simulink model "UDPMain_MoveToPoint"  (R2022a)
settings: Solver=FixedStepAuto  StartTime=0.0  StopTime=inf  FixedStep=1/model_frequency  RelTol=1e-3
values from neighbouring files (symbols this model uses):
  markers = [markers;i]    [loadMapData.m]
  send_data_length = num_floats_to_send*4    (= 12)    [initUDP.m]
  steerLim = [-40,40]    [initUDP.m]
  velLim = [-2,5]    [initUDP.m]
libraries: slrealtimeutilitieslib x2, slrealtimeiplib x2, simulink_extras x1
settings Model: Creator=aljaz  LastModifiedBy=aljaz
settings SolverCC: AlgebraicLoopSolver=TrustRegion
settings DebuggingCC: UnconnectedInputMsg=warning  UnconnectedOutputMsg=warning  UnconnectedLineMsg=warning  SFMachineParentedDataDiag=warning
settings RTWCC: DLArmComputeVersion=19.05

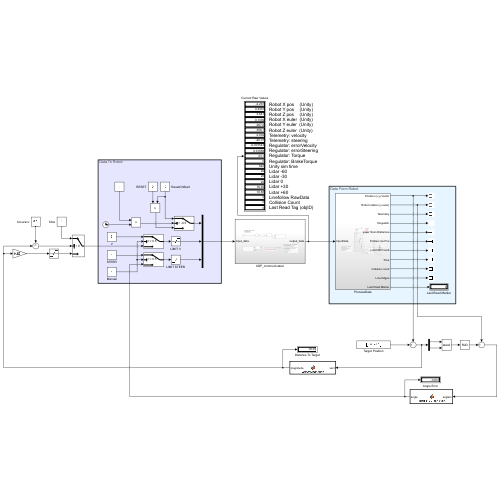
[thumbnail: Simulink's stored preview of the top-level diagram]
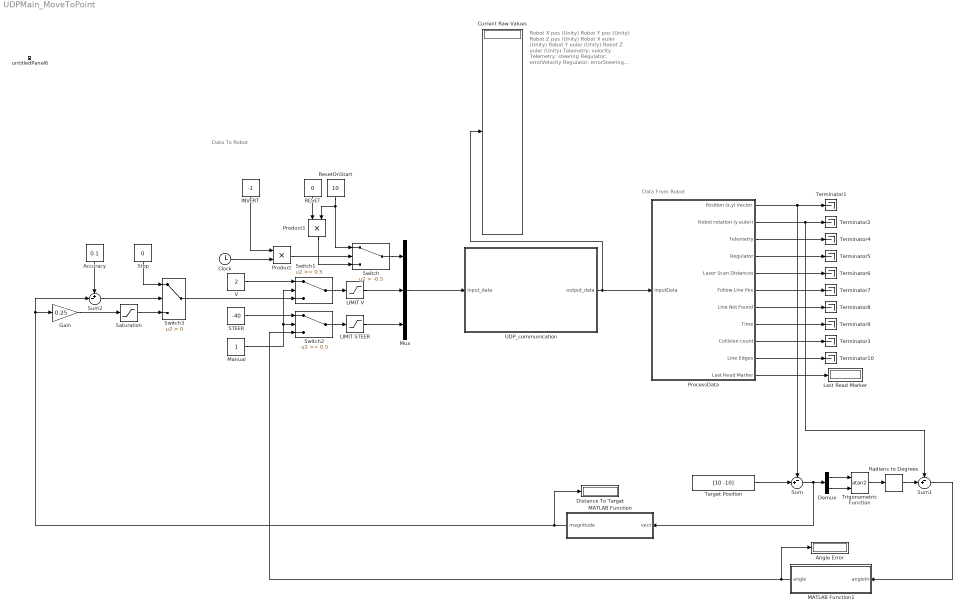
== system UDPMain_MoveToPoint ==
  note: Data From Robot
  note: Data To Robot
  note: Robot X pos (Unity)
      | Robot Y pos (Unity)
      | Robot Z pos (Unity)
      | Robot X euler (Unity)
      | Robot Y euler (Unity)
      | Robot Z euler (Unity)
      | Telemetry: velocity
      | Telemetry: steering
      | Regulator: errorVelocity
      | Regulator: errorSteering
      | Regulator: Torque
      | Regulator: BrakeTorque
      | Unity sim time
      | Lidar -60
      | Lidar -30
      | Lidar 0
      | Lidar +30
      | Lidar +60
      | Linefollow RawData
      | Collision Count
      | Last Read Tag (objID)
  Accuracy : Constant  Value=0.1
  Angle Error : Display
  Clock : Clock
  Current Raw Values : Display
  Demux : Demux  Outputs=2
  Distance To Target : Display
  Gain : Gain  Gain=0.25
  INVERT : Constant  Value=-1
  LIMIT STEER : Saturate  UpperLimit=steerLim(2)  LowerLimit=steerLim(1)
  LIMIT V : Saturate  UpperLimit=velLim(2)  LowerLimit=velLim(1)
  Last Read Marker : Display
  MATLAB Function : MATLAB Function  TreatAsAtomicUnit=on
  MATLAB Function1 : MATLAB Function  TreatAsAtomicUnit=on
  Manual : Constant
  Mux : Mux  Inputs=3
  ProcessData : Subsystem
  Product : Product
  Product1 : Product
  RESET : Constant  Value=0
  Radians to Degrees : simulink_extras/Transformations/Radians to Degrees
  ResetOnStart : Constant  Value=10
  STEER : Constant  Value=-40
  Saturation : Saturate  UpperLimit=1  LowerLimit=-1
  Stop : Constant  Value=0
  Sum : Sum  Inputs=-+|
  Sum1 : Sum  Inputs=-+|
  Sum2 : Sum  Inputs=+-|
  Switch : Switch  Criteria=u2 > Threshold  Threshold=-0.5  SaturateOnIntegerOverflow=off  InputSameDT=off
  Switch1 : Switch  Threshold=0.5  SaturateOnIntegerOverflow=off  InputSameDT=off
  Switch2 : Switch  Threshold=0.5  SaturateOnIntegerOverflow=off  InputSameDT=off
  Switch3 : Switch  Criteria=u2 > Threshold  SaturateOnIntegerOverflow=off  InputSameDT=off
  Target Position : Constant  Value=[10 -10]
  Terminator{1..10} (10 alike) : Terminator
  Trigonometric Function : Trigonometry  Operator=atan2
  UDP_communication : Subsystem
  V : Constant  Value=2
  untitledPanel6 : Subsystem  Tag=HiddenForWebPanel  IsWebBlockPanel=on
  wires:
  UDP_communication/1(output_data) -> Current Raw Values/1, ProcessData/1(InputData)
  ProcessData/9(Collision count) -> Terminator3/1
  ProcessData/2(Robot rotation (y euler)) -> Terminator2/1, Sum1/1
  ProcessData/1(Position (x,y) Vector) -> Sum/1, Terminator1/1
  Mux/1 -> UDP_communication/1(input_data)
  INVERT/1 -> Product/1
  Product/1 -> Switch/2
  Clock/1 -> Product/2
  Switch/1 -> Mux/1
  RESET/1 -> Product1/1
  LIMIT V/1 -> Mux/2
  LIMIT STEER/1 -> Mux/3
  Switch1/1 -> LIMIT V/1
  V/1 -> Switch1/1
  Manual/1 -> Switch2/2, Switch1/2
  Switch2/1 -> LIMIT STEER/1
  STEER/1 -> Switch2/1
  ProcessData/3(Telemetry) -> Terminator4/1
  ProcessData/4(Regulator) -> Terminator5/1
  ProcessData/5(Laser Scan Distances) -> Terminator6/1
  ProcessData/6(Follow Line Pos) -> Terminator7/1
  ProcessData/7(Line Not Found) -> Terminator8/1
  ProcessData/8(Time) -> Terminator9/1
  ResetOnStart/1 -> Switch/1, Product1/2
  Product1/1 -> Switch/3
  ProcessData/11(Last Read Marker) -> Last Read Marker/1
  ProcessData/10(Line Edges) -> Terminator10/1
  Sum1/1 -> MATLAB Function1/1(angleIn)
  Target Position/1 -> Sum/2
  Sum/1 -> MATLAB Function/1(vect), Demux/1
  Demux/1 -> Trigonometric Function/1
  Demux/2 -> Trigonometric Function/2
  Trigonometric Function/1 -> Radians to Degrees/1
  MATLAB Function/1(magnitude) -> Sum2/2, Gain/1, Distance To Target/1
  Gain/1 -> Saturation/1
  Radians to Degrees/1 -> Sum1/2
  Switch3/1 -> Switch1/3
  Sum2/1 -> Switch3/2
  Saturation/1 -> Switch3/3
  Stop/1 -> Switch3/1
  Accuracy/1 -> Sum2/1
  MATLAB Function1/1(angle) -> Switch2/3, Angle Error/1

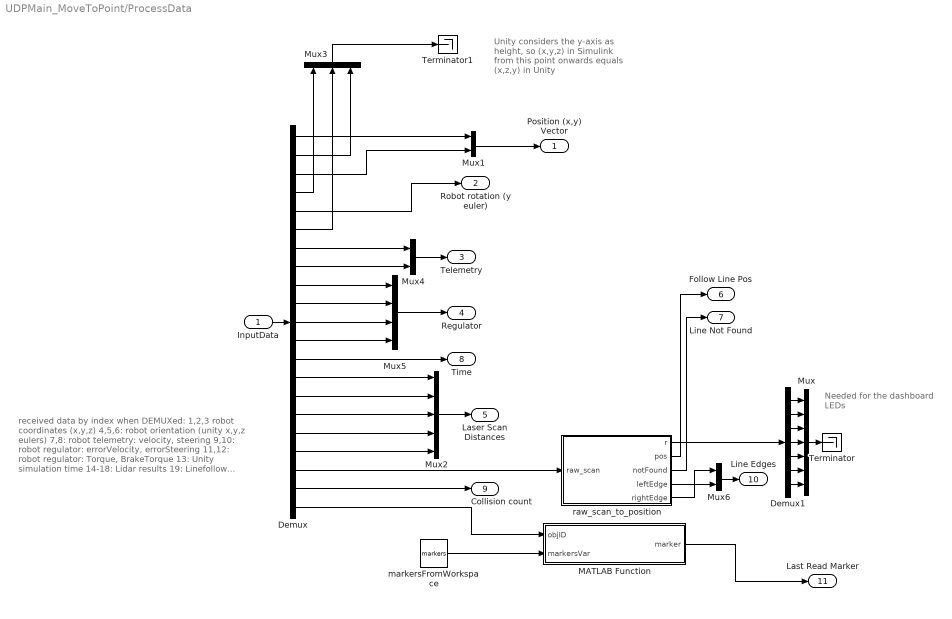
== system UDPMain_MoveToPoint/ProcessData ==
  note: Unity considers the y-axis as height, so (x,y,z) in Simulink from this point onwards equals (x,z,y) in Unity
  note: Needed for the dashboard LEDs
  note: received data by index when DEMUXed:
      | 1,2,3 robot coordinates (x,y,z)
      | 4,5,6: robot orientation (unity x,y,z eulers)
      | 7,8: robot telemetry: velocity, steering
      | 9,10: robot regulator: errorVelocity, errorSteering
      | 11,12: robot regulator: Torque, BrakeTorque
      | 13: Unity simulation time
      | 14-18: Lidar results
      | 19: Linefollow binary results
  InputData : Inport
  Demux : Demux  Outputs=21
  Demux1 : Demux  Outputs=7
  MATLAB Function : MATLAB Function  TreatAsAtomicUnit=on
  Mux : Mux  Inputs=7
  Mux1 : Mux  Inputs=2
  Mux2 : Mux  Inputs=5
  Mux3 : Mux  Inputs=3
  Mux4 : Mux  Inputs=2
  Mux5 : Mux
  Mux6 : Mux  Inputs=2
  Terminator : Terminator
  Terminator1 : Terminator
  markersFromWorkspace : Constant  Value=markers
  raw_scan_to_position : MATLAB Function  TreatAsAtomicUnit=on
  Position (x,y) Vector : Outport
  Robot rotation (y euler) : Outport  Port=2
  Telemetry : Outport  Port=3
  Regulator : Outport  Port=4
  Laser Scan Distances : Outport  Port=5
  Follow Line Pos : Outport  Port=6
  Line Not Found : Outport  Port=7
  Time : Outport  Port=8
  Collision count : Outport  Port=9
  Line Edges : Outport  Port=10
  Last Read Marker : Outport  Port=11
  wires:
  InputData/1 -> Demux/1
  Demux/1 -> Mux1/1
  Mux1/1 -> Position (x,y) Vector/1
  Demux/20 -> Collision count/1
  raw_scan_to_position/2(pos) -> Follow Line Pos/1
  raw_scan_to_position/1(r) -> Demux1/1
  Demux1/4 -> Mux/4
  Demux1/1 -> Mux/1
  Demux1/2 -> Mux/2
  Demux1/3 -> Mux/3
  Demux1/5 -> Mux/5
  Demux1/6 -> Mux/6
  Demux1/7 -> Mux/7
  Mux/1 -> Terminator/1
  raw_scan_to_position/3(notFound) -> Line Not Found/1
  Mux2/1 -> Laser Scan Distances/1
  Demux/3 -> Mux1/2
  Demux/2 -> Mux3/3
  Demux/5 -> Robot rotation (y euler)/1
  Mux3/1 -> Terminator1/1
  Demux/4 -> Mux3/1
  Demux/6 -> Mux3/2
  Demux/14 -> Mux2/1
  Demux/15 -> Mux2/2
  Demux/16 -> Mux2/3
  Demux/17 -> Mux2/4
  Demux/18 -> Mux2/5
  Demux/19 -> raw_scan_to_position/1(raw_scan)
  Demux/7 -> Mux4/1
  Demux/8 -> Mux4/2
  Mux4/1 -> Telemetry/1
  Demux/9 -> Mux5/1
  Demux/10 -> Mux5/2
  Demux/11 -> Mux5/3
  Demux/12 -> Mux5/4
  Mux5/1 -> Regulator/1
  Demux/13 -> Time/1
  Mux6/1 -> Line Edges/1
  raw_scan_to_position/5(rightEdge) -> Mux6/1
  raw_scan_to_position/4(leftEdge) -> Mux6/2
  Demux/21 -> MATLAB Function/1(objID)
  MATLAB Function/1(marker) -> Last Read Marker/1
  markersFromWorkspace/1 -> MATLAB Function/2(markersVar)

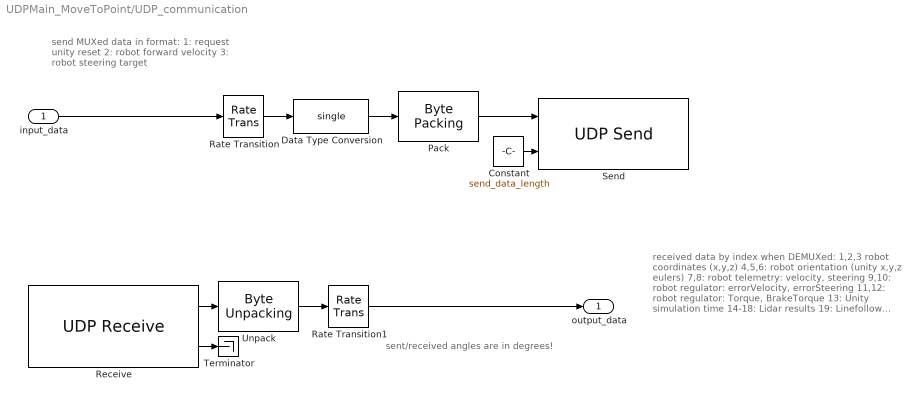
== system UDPMain_MoveToPoint/UDP_communication ==
  note: sent/received angles are in degrees!
  note: send MUXed data in format:
      | 1: request unity reset
      | 2: robot forward velocity
      | 3: robot steering target
  note: received data by index when DEMUXed:
      | 1,2,3 robot coordinates (x,y,z)
      | 4,5,6: robot orientation (unity x,y,z eulers)
      | 7,8: robot telemetry: velocity, steering
      | 9,10: robot regulator: errorVelocity, errorSteering
      | 11,12: robot regulator: Torque, BrakeTorque
      | 13: Unity simulation time
      | 14-18: Lidar results
      | 19: Linefollow binary results
      | 20: Collision count
      | 21: last read Tag
  input_data : Inport
  Constant : Constant  Value=send_data_length
  Data Type Conversion : DataTypeConversion  OutDataTypeStr=single  SaturateOnIntegerOverflow=off  RndMeth=Floor
  Pack : slrealtimeutilitieslib/Byte Packing  MaskPackedDataType=uint8  MaskUnpackedDataTypes={'single'}  MaskAlignment=1
  Rate Transition : RateTransition
  Rate Transition1 : RateTransition
  Receive : slrealtimeiplib/UDP Receive  useHostTargetConn=on  ipAddress=10.10.10.15  localPort=25106  rcvWidth=receive_data_length  rcvFmAny=off  fmAddress=127.0.0.1  sampleTime=0.01  enableMessage=off  maxPackets=1
      settings: SourceProductBaseCode=XP
  Send : slrealtimeiplib/UDP Send  useHostTargetConn=on  toAddress=127.0.0.1  toPort=25008  sampleTime=0.01  enableMessage=off  ipAddress=10.10.10.15  localPort=-1
      settings: SourceProductBaseCode=XP
  Terminator : Terminator
  Unpack : slrealtimeutilitieslib/Byte Unpacking  MaskUnpackedDataTypes={'single'}  MaskUnpackedDataSizes={[num_floats_to_receive]}  MaskAlignment=1
      settings: SourceProductBaseCode=XP
  output_data : Outport
  wires:
  Rate Transition1/1 -> output_data/1
  Unpack/1 -> Rate Transition1/1
  Rate Transition/1 -> Data Type Conversion/1
  Receive/1 -> Unpack/1
  Constant/1 -> Send/2
  Receive/2 -> Terminator/1
  Pack/1 -> Send/1
  Data Type Conversion/1 -> Pack/1
  input_data/1 -> Rate Transition/1

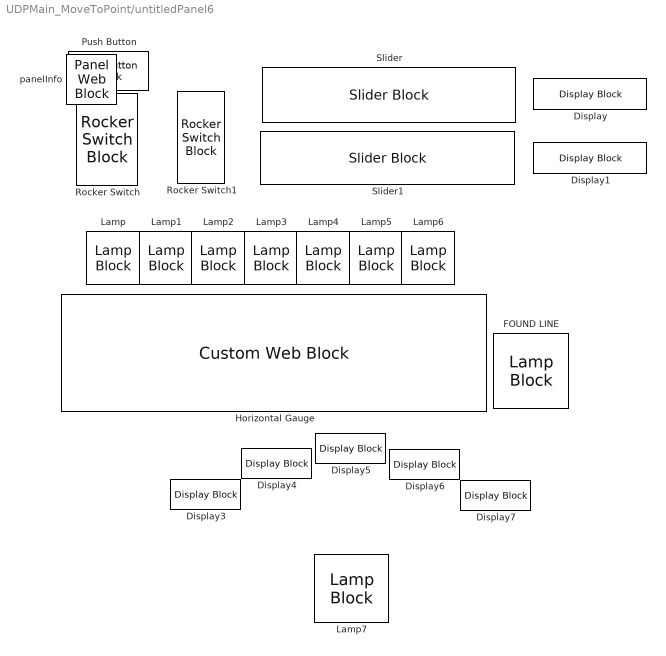
== system UDPMain_MoveToPoint/untitledPanel6 ==
  Display : DisplayBlock  Tag=HiddenForWebPanel  PanelInfo="{\"panelId\":\"panelId-3b0286ef-9598-43d7-b16e-0edae3a5bc45\",\"type\":\"panelChild\",\"version\":\"2019b\",\"zIndex\":1500028}"  LabelPosition=Hide  Transparency=1
  Display1 : DisplayBlock  Tag=HiddenForWebPanel  PanelInfo="{\"panelId\":\"panelId-3b0286ef-9598-43d7-b16e-0edae3a5bc45\",\"type\":\"panelChild\",\"version\":\"2019b\",\"zIndex\":1500030}"  LabelPosition=Hide  Transparency=1
  Display3 : DisplayBlock  Tag=HiddenForWebPanel  PanelInfo="{\"panelId\":\"panelId-3b0286ef-9598-43d7-b16e-0edae3a5bc45\",\"type\":\"panelChild\",\"version\":\"2019b\",\"zIndex\":1500034}"  LabelPosition=Hide  Transparency=1
  Display4 : DisplayBlock  Tag=HiddenForWebPanel  PanelInfo="{\"panelId\":\"panelId-3b0286ef-9598-43d7-b16e-0edae3a5bc45\",\"type\":\"panelChild\",\"version\":\"2019b\",\"zIndex\":1500036}"  LabelPosition=Hide  Transparency=1
  Display5 : DisplayBlock  Tag=HiddenForWebPanel  PanelInfo="{\"panelId\":\"panelId-3b0286ef-9598-43d7-b16e-0edae3a5bc45\",\"type\":\"panelChild\",\"version\":\"2019b\",\"zIndex\":1500038}"  LabelPosition=Hide  Transparency=1
  Display6 : DisplayBlock  Tag=HiddenForWebPanel  PanelInfo="{\"panelId\":\"panelId-3b0286ef-9598-43d7-b16e-0edae3a5bc45\",\"type\":\"panelChild\",\"version\":\"2019b\",\"zIndex\":1500040}"  LabelPosition=Hide  Transparency=1
  Display7 : DisplayBlock  Tag=HiddenForWebPanel  PanelInfo="{\"panelId\":\"panelId-3b0286ef-9598-43d7-b16e-0edae3a5bc45\",\"type\":\"panelChild\",\"version\":\"2019b\",\"zIndex\":1500042}"  LabelPosition=Hide  Transparency=1
  FOUND LINE : LampBlock  Tag=HiddenForWebPanel  PanelInfo="{\"panelId\":\"panelId-3b0286ef-9598-43d7-b16e-0edae3a5bc45\",\"type\":\"panelChild\",\"version\":\"2019b\",\"zIndex\":1500004}"
  Horizontal Gauge : CustomWebBlock  Tag=HiddenForWebPanel  PanelInfo="{\"panelId\":\"panelId-3b0286ef-9598-43d7-b16e-0edae3a5bc45\",\"type\":\"panelChild\",\"version\":\"2019b\",\"zIndex\":1500002}"  ShowInitialText=on  Configuration="{\"type\":\"LinearGauge\",\"settings\":{\"BindingType\":\"signal\",\"aspectRatio\":3.7578947368421054,\"fixedAspectRatio\":\"on\",\"orientation\":\"horizontal\"},\"components\":[{\"name\":\"LinearScaleComponent\",\"settings\":{\"bounds\":{\"max\":0.3,\"min\":-0.3,\"tickInterval\":\"auto\"},\"internalTickHeightScaleFactor\":0.5,\"labelColor\":[250,245,199],\"labelFont\":{\"font\":\"Arial\",\"fontSize\":12},\"labelTransparency\":1,\"needleImage\":{\"size\":[21,75],\"src\":\"data:image/svg+xml;base64,PHN2ZyB4bWxucz0iaHR0cDovL3d3dy53My5vcmcvMjAwMC9zdmciIHhtbG5zOnhsaW5rPSJodHRwOi8vd3d3LnczLm9yZy8xOTk5L3hsaW5rIiB2aWV3Qm94PSIwIDAgMjEgNzUiPjxkZWZzPjxzdHlsZT4uY2xzLTF7ZmlsbDpub25lO30uY2xzLTJ7aXNvbGF0aW9uOmlzb2xhdGU7fS5jbHMtM3tjbGlwLXBhdGg6dXJsKCNjbGlwLXBhdGgpO30uY2xzLTR7b3BhY2l0eTowLjM7bWl4LWJsZW5kLW1vZGU6bXVsdGlwbHk7fS5jbHMtNXtmaWxsOiNlYjI2Mjk7fTwvc3R5bGU+PGNsaXBQYXRoIGlkPSJjbGlwLXBhdGgiIHRyYW5zZm9y ...(+1928 chars)\",\"srcOrientation\":\"horizontal\"},\"needleOffset\":[0,0.01094391244870041],\"needleSize\":{\"height\":0.7589285714285714,\"width\":0.11960078534031414},\"position\":[0.06986607142857143,0.01995798319327731,0.9641544117647058,0.8],\"referencePoint\":\"auto\",\"scaleColors\":[],\"scaleColorsSize\":0.2,\"scaleDirection\":\"LR\",\"showLabels\":1,\"showMinorTicks\":0,\"showSpanLine\":1,\"showTicks\":1,\"tickColor\":[250,245,200],\"tickTransparency\":1,\"valueBarColor\":[23,89,176],\"valueBarOffset\":0,\"valueBarSize\":0.23,\"valueBarTransparency\":1}},{\"name\":\"BackgroundImageComponent\",\"settings\":{\"image\":{\"size\":[380,101],\"src\":\"data:image/svg+xml;base64,PHN2ZyB4bWxucz0iaHR0cDovL3d3dy53My5vcmcvMjAwMC9zdmciIHZpZXdCb3g9IjAgMCAzODAgMTAxIj48ZGVmcz48c3R5bGU+LmNscy0xe2ZpbGw6IzAwMmI0Mjt9LmNscy0ye2ZpbGw6IzQyNzA4Mjt9LmNscy0ze2ZpbGw6IzdjYTBiMjt9PC9zdHlsZT48L2RlZnM+PHRpdGxlPmhvcml6b250YWxfZ2F1Z2VfIGJhY2tncm91bmQ8L3RpdGxlPjxnIGlkPSJMYXllcl8yIiBkYXRhLW5hbWU9IkxheWVyIDIiPjxnIGlkPSJMYXllcl8xLTIiIGRhdGEtbmFtZT0iTGF5ZXIgMSI+PHJlY3QgY2xhc3M9ImNscy0xIiB4PSIxMSIgeT0iMTEiIHdpZHRoPSIzNTgiIGhlaWdodD0iNzkiLz48cGF0aCBjbGFzcz0iY2xzLTIiIGQ9Ik04LDhWOTNIMzcyVjhaTTM2OSw5MEgxMVYxMUgzNjlaIi8+PHBhdGggY2xhc3M9ImNscy0zIiBkPSJNMCwwVjEwMUgzODBWMFpNMzcyLDkzSDhWOEgzNzJaIi8+PC9nPjwvZz48L3N2Zz4=\",\"srcOrientation\":\"horizontal\"},\"position\":[0,0,1,1],\"scaleMode\":\"0\"}},{\"name\":\"ForegroundImageComponent\",\"settings\":{\"image\":{\"size\":[0,0],\"src\":\"default\",\"srcOrientation\":[]},\"isForeground\":1,\"position\":[0,0,1,1],\"scaleMode\":\"0\"}}]}"
  Lamp : LampBlock  Tag=HiddenForWebPanel  PanelInfo="{\"panelId\":\"panelId-3b0286ef-9598-43d7-b16e-0edae3a5bc45\",\"type\":\"panelChild\",\"version\":\"2019b\",\"zIndex\":1500006}"
  Lamp1 : LampBlock  Tag=HiddenForWebPanel  PanelInfo="{\"panelId\":\"panelId-3b0286ef-9598-43d7-b16e-0edae3a5bc45\",\"type\":\"panelChild\",\"version\":\"2019b\",\"zIndex\":1500008}"
  Lamp2 : LampBlock  Tag=HiddenForWebPanel  PanelInfo="{\"panelId\":\"panelId-3b0286ef-9598-43d7-b16e-0edae3a5bc45\",\"type\":\"panelChild\",\"version\":\"2019b\",\"zIndex\":1500010}"
  Lamp3 : LampBlock  Tag=HiddenForWebPanel  PanelInfo="{\"panelId\":\"panelId-3b0286ef-9598-43d7-b16e-0edae3a5bc45\",\"type\":\"panelChild\",\"version\":\"2019b\",\"zIndex\":1500012}"
  Lamp4 : LampBlock  Tag=HiddenForWebPanel  PanelInfo="{\"panelId\":\"panelId-3b0286ef-9598-43d7-b16e-0edae3a5bc45\",\"type\":\"panelChild\",\"version\":\"2019b\",\"zIndex\":1500014}"
  Lamp5 : LampBlock  Tag=HiddenForWebPanel  PanelInfo="{\"panelId\":\"panelId-3b0286ef-9598-43d7-b16e-0edae3a5bc45\",\"type\":\"panelChild\",\"version\":\"2019b\",\"zIndex\":1500016}"
  Lamp6 : LampBlock  Tag=HiddenForWebPanel  PanelInfo="{\"panelId\":\"panelId-3b0286ef-9598-43d7-b16e-0edae3a5bc45\",\"type\":\"panelChild\",\"version\":\"2019b\",\"zIndex\":1500018}"
  Lamp7 : LampBlock  Tag=HiddenForWebPanel  PanelInfo="{\"panelId\":\"panelId-3b0286ef-9598-43d7-b16e-0edae3a5bc45\",\"type\":\"panelChild\",\"version\":\"2019b\",\"zIndex\":1500048}"  LabelPosition=Hide
  Push Button : PushButtonBlock  Tag=HiddenForWebPanel  PanelInfo="{\"panelId\":\"panelId-3b0286ef-9598-43d7-b16e-0edae3a5bc45\",\"type\":\"panelChild\",\"version\":\"2019b\",\"zIndex\":1500022}"  ButtonText=RESET  OffValue=0.000000
  Rocker Switch : RockerSwitchBlock  Tag=HiddenForWebPanel  PanelInfo="{\"panelId\":\"panelId-3b0286ef-9598-43d7-b16e-0edae3a5bc45\",\"type\":\"panelChild\",\"version\":\"2019b\",\"zIndex\":1500020}"
      settings: Values={{'Off', 'On'}, [0 1]}
  Rocker Switch1 : RockerSwitchBlock  Tag=HiddenForWebPanel  PanelInfo="{\"panelId\":\"panelId-3b0286ef-9598-43d7-b16e-0edae3a5bc45\",\"type\":\"panelChild\",\"version\":\"2019b\",\"zIndex\":1500046}"
      settings: Values={{'Off', 'On'}, [0 1]}
  Slider : SliderBlock  Tag=HiddenForWebPanel  PanelInfo="{\"panelId\":\"panelId-3b0286ef-9598-43d7-b16e-0edae3a5bc45\",\"type\":\"panelChild\",\"version\":\"2019b\",\"zIndex\":1500024}"  ScaleMin=-2  ScaleMax=5  TickInterval=0.5
  Slider1 : SliderBlock  Tag=HiddenForWebPanel  PanelInfo="{\"panelId\":\"panelId-3b0286ef-9598-43d7-b16e-0edae3a5bc45\",\"type\":\"panelChild\",\"version\":\"2019b\",\"zIndex\":1500026}"  ScaleMin=-40  ScaleMax=40  TickInterval=20
  panelInfo : PanelWebBlock  Tag=HiddenForWebPanel  PanelInfo="{\"compacted\":false,\"height\":619,\"isActiveTab\":true,\"labels\":{\"label2777103104\":{\"left\":\"434\",\"settings\":{\"backgroundColor\":\"rgba(0, 0, 0, 0)\",\"bold\":true,\"font\":\"Arial\",\"fontColor\":\"black\",\"fontSize\":0.9,\"italicized\":false,\"underlined\":false},\"text\":\"LINE FOUND?\",\"top\":\"270\"},\"label4548952663\":{\"left\":\"178\",\"settings\":{\"backgroundColor\":\"rgba(0, 0, 0, 0)\",\"bold\":true,\"font\":\"Arial\",\"fontColor\":\"black\",\"fontSize\":1,\"italicized\":false,\"underlined\":false},\"text\":\"\\nLASER SCANNER\\n(30 deg step)\",\"top\":\"475\"},\"label5306036013\":{\"left\":\"483\",\"settings\":{\"backgroundColor\":\"rgba(0, 0, 0, 0)\",\"bold\":true,\"font\":\"Arial\",\"fontColor\":\"black\",\"fontSize\":1,\"italicized\":false,\"underlined\":false},\"text\":\"sent Velocity\",\"top\":\"16\"},\"label6759266376\":{\"left\":\"484\",\"settings\":{\"backgroundColor\":\"rgba(0, 0, 0, 0)\",\"bold\":true,\"font\":\"Arial\",\"fontColor\":\"black\",\"fontSize\":1,\"italicized\":false,\"underlined\":false},\"text\":\"sent Steer\",\"top\":\"81\"},\"label7063265318\":{\"left\":\"258\",\"settings\":{\"backgroundColor\":\"rgba(0, 0, 0, 0)\",\"bold\":true,\"font\":\"Arial\",\"fontColor\":\"black\",\"fontSize\":0.9,\"italicized\":false,\"underlined\":false},\"text\":\"COLLISION?\",\"top\":\"582\"},\"label7981171109\":{\"left\":\"102\",\"settings\":{\"backgroundColor\":\"rgba(0, 0, 0, 0)\",\"bold\":false,\"font\":\"Arial\",\"fontColor\":\"black\",\"fontSize\":0.9,\"italicized\":false,\"underlined\":false},\"text\":\"Manual Control\",\"top\":\"35\"},\"label9223960395\":{\"left\":\"166\",\"settings\":{\"backgroundColor\":\"rgba(0, 0, 0, 0)\",\"bold\":true,\"font\":\"Arial\",\"fontColor\":\"black\",\"fontSize\":1,\"italicized\":false,\"underlined\":false},\"text\":\"FOLLOW LINE\",\"top\":\"164\"}},\"left\":-12,\"name\":\"untitledPanel2\",\"panelId\":\"panelId-3b0286ef-9598-43d7-b16e-0edae3a5bc45\",\"tabIndex\":0,\"tabbedSetId\":\"tabbedSet4971406738\",\"top\":2,\"type\":\"panel\",\"version\":\"2019b\",\"visible\":true,\"width\":615,\"zIndex\":1500014}"  PanelSnapshot=<binary blob, 82268 chars, not shown>

== matlab function UDPMain_MoveToPoint/MATLAB Function ==
  data: vect input; magnitude output
function magnitude=VectorMagnitude(vect)
magnitude=sqrt(vect(1)*vect(1)+vect(2)*vect(2));

== matlab function UDPMain_MoveToPoint/ProcessData/raw_scan_to_position ==
  data: raw_scan input; r output size=[1,7]; pos output size=1; rayDistance parameter; notFound output; leftEdge output; rightEdge output
function [r,pos,notFound,leftEdge,rightEdge] = fcn(raw_scan,rayDistance)
leftEdge=0;
rightEdge=0;
raw_scan=round(raw_scan);
result=arrayfun(@(x) mod(floor(raw_scan/10^x),10),floor(log10(raw_scan)):-1:0);
if length(result)<7
    tempZeros=zeros(1,7-length(result));
    result=[tempZeros,result];
end
r=zeros(1,7);
pos=0;
count=0;

for ii=1:7
    r(ii)=result(ii);
    currPos=(-4+ii)*rayDistance;
    pos=pos+r(ii)*currPos;
    count=count+r(ii);
    if (r(ii)~=0)
        if (count==1)
            leftEdge=currPos;
        end
        rightEdge=currPos;
    end
end
if count>0
    pos=pos/count;
end
if count==0
    notFound=1;
else
    notFound=0;
end

== matlab function UDPMain_MoveToPoint/MATLAB Function1 ==
  data: angleIn input; angle output
function angle=Handle180Transition(angleIn)

angle=angleIn;
if (angleIn>180)
    angle=angleIn-360;
end
if (angleIn<-180)
    angle=angleIn+360;
end

== matlab function UDPMain_MoveToPoint/ProcessData/MATLAB Function ==
  data: objID input; marker output; markersVar input
function marker=getTagID(objID,markersVar)
marker=0;
for ii=1:size(markersVar,1)
    if (markersVar(ii)==objID)
       marker=ii+1;
       break;
    end
end
